simulink model "trajectory_IMU"  (R2021a)
settings: Solver=VariableStepAuto  StartTime=0.0  StopTime=tf  RelTol=1e-3
settings Model: Creator=Laura  LastModifiedBy=Laura

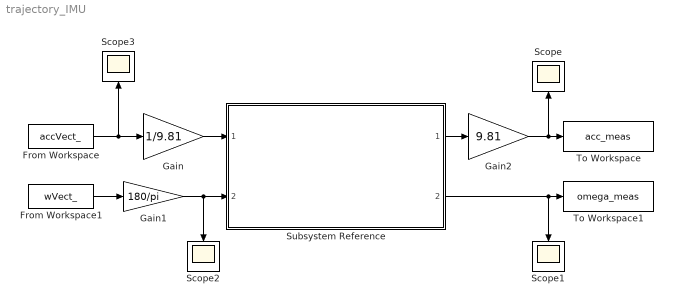
== system trajectory_IMU ==
  From Workspace : FromWorkspace  VariableName=accVect_
  From Workspace1 : FromWorkspace  VariableName=wVect_
  Gain : Gain  Gain=1/9.81
  Gain1 : Gain  Gain=180/pi
  Gain2 : Gain  Gain=9.81
  Scope{,1..3} (4 alike) : Scope
  Subsystem Reference : Subsystem  ReferencedSubsystem=IMU
  To Workspace : ToWorkspace  VariableName=acc_meas  SaveFormat=Timeseries  SampleTime=-1
  To Workspace1 : ToWorkspace  VariableName=omega_meas  SaveFormat=Timeseries  SampleTime=-1
  wires:
  Subsystem Reference/1 -> Gain2/1
  From Workspace1/1 -> Gain1/1
  From Workspace/1 -> Scope3/1, Gain/1
  Gain/1 -> Subsystem Reference/1
  Gain2/1 -> Scope/1, To Workspace/1
  Subsystem Reference/2 -> To Workspace1/1, Scope1/1
  Gain1/1 -> Scope2/1, Subsystem Reference/2
